simulink model "HardwareControlSample"  (R2015a)
settings: configuration reference "SIMULATION_CONFIGURATION" (kept outside this file)
settings Model: Creator=moritz  LastModifiedBy=moritz
settings ConfigSetRef: SourceLocation=Base Workspace

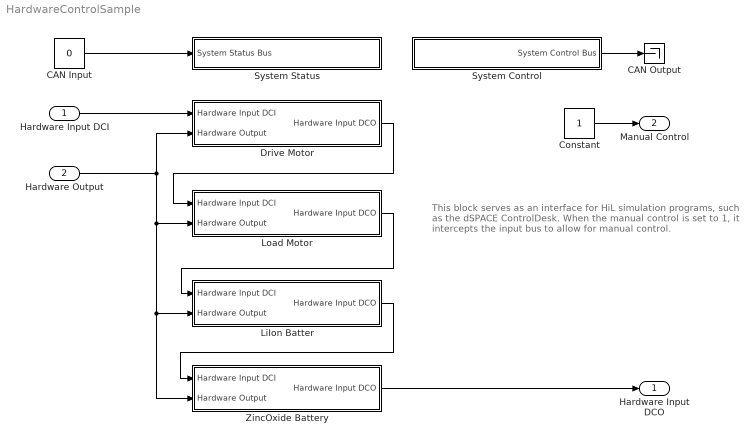
== system HardwareControlSample ==
  note: This block serves as an interface for HiL simulation programs, such as the dSPACE ControlDesk. When the manual control is set to 1, it intercepts the input bus to allow for manual control.
  Hardware Input DCI : Inport  OutDataTypeStr=Bus: HARDWARE_INPUT_BUS  BusOutputAsStruct=on
  Hardware Output : Inport  Port=2  OutDataTypeStr=Bus: HARDWARE_OUTPUT_BUS  BusOutputAsStruct=on
  CAN Input : Constant  Value=0  OutDataTypeStr=Inherit: Inherit via back propagation
  CAN Output : Terminator
  Constant : Constant  OutDataTypeStr=boolean
  Drive Motor : Subsystem
  LiIon Batter : Subsystem
  Load Motor : Subsystem
  System Control : Subsystem
  System Status : Subsystem
  ZincOxide Battery : Subsystem
  Hardware Input DCO : Outport  OutDataTypeStr=Bus: HARDWARE_INPUT_BUS  BusOutputAsStruct=on
  Manual Control : Outport  Port=2
  wires:
  Constant/1 -> Manual Control/1
  Hardware Input DCI/1 -> Drive Motor/1(Hardware Input DCI)
  Hardware Output/1 -> ZincOxide Battery/2(Hardware Output), LiIon Batter/2(Hardware Output), Load Motor/2(Hardware Output), Drive Motor/2(Hardware Output)
  Drive Motor/1(Hardware Input DCO) -> Load Motor/1(Hardware Input DCI)
  Load Motor/1(Hardware Input DCO) -> LiIon Batter/1(Hardware Input DCI)
  LiIon Batter/1(Hardware Input DCO) -> ZincOxide Battery/1(Hardware Input DCI)
  ZincOxide Battery/1(Hardware Input DCO) -> Hardware Input DCO/1
  System Control/1(System Control Bus) -> CAN Output/1
  CAN Input/1 -> System Status/1(System Status Bus)

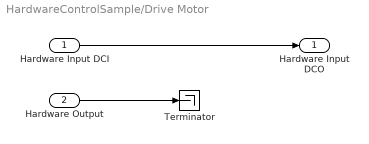
== system HardwareControlSample/Drive Motor ==
  Hardware Input DCI : Inport
  Hardware Output : Inport  Port=2
  Terminator : Terminator
  Hardware Input DCO : Outport
  wires:
  Hardware Input DCI/1 -> Hardware Input DCO/1
  Hardware Output/1 -> Terminator/1

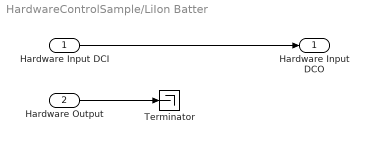
== system HardwareControlSample/LiIon Batter ==
  Hardware Input DCI : Inport
  Hardware Output : Inport  Port=2
  Terminator : Terminator
  Hardware Input DCO : Outport
  wires:
  Hardware Input DCI/1 -> Hardware Input DCO/1
  Hardware Output/1 -> Terminator/1

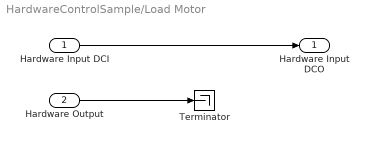
== system HardwareControlSample/Load Motor ==
  Hardware Input DCI : Inport
  Hardware Output : Inport  Port=2
  Terminator : Terminator
  Hardware Input DCO : Outport
  wires:
  Hardware Input DCI/1 -> Hardware Input DCO/1
  Hardware Output/1 -> Terminator/1

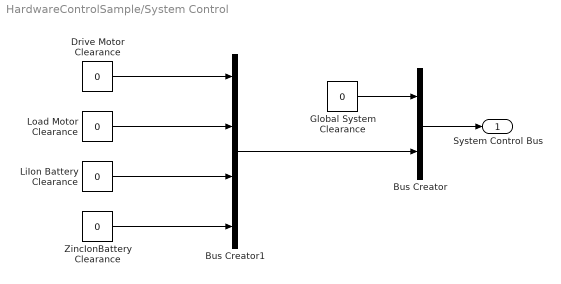
== system HardwareControlSample/System Control ==
  Bus Creator : BusCreator  Inputs=2
  Bus Creator1 : BusCreator
  Drive Motor Clearance : Constant  Value=0  OutDataTypeStr=boolean
  Global System Clearance : Constant  Value=0  OutDataTypeStr=boolean
  LiIon Battery Clearance : Constant  Value=0  OutDataTypeStr=boolean
  Load Motor Clearance : Constant  Value=0  OutDataTypeStr=boolean
  ZincIonBattery Clearance : Constant  Value=0  OutDataTypeStr=boolean
  System Control Bus : Outport
  wires:
  Bus Creator/1 -> System Control Bus/1
  Global System Clearance/1 -> Bus Creator/1
  Bus Creator1/1 -> Bus Creator/2
  Drive Motor Clearance/1 -> Bus Creator1/1
  Load Motor Clearance/1 -> Bus Creator1/2
  LiIon Battery Clearance/1 -> Bus Creator1/3
  ZincIonBattery Clearance/1 -> Bus Creator1/4

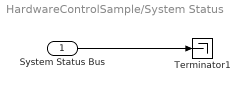
== system HardwareControlSample/System Status ==
  System Status Bus : Inport
  Terminator1 : Terminator
  wires:
  System Status Bus/1 -> Terminator1/1

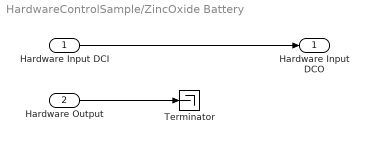
== system HardwareControlSample/ZincOxide Battery ==
  Hardware Input DCI : Inport
  Hardware Output : Inport  Port=2
  Terminator : Terminator
  Hardware Input DCO : Outport
  wires:
  Hardware Input DCI/1 -> Hardware Input DCO/1
  Hardware Output/1 -> Terminator/1
